simulink model "part2_MAIN"  (R2023b)
settings: Solver=FixedStepAuto  StartTime=0.0  StopTime=300  FixedStep=0.1  RelTol=1e-3
values from neighbouring files (symbols this model uses):
  Af = diag(ti)    [init.m]
  Aw = [zeros(3) eye(3) ... (first row only)    [get_observer_parameters.m]
  B = [zeros(6,3);zeros(3,3);zeros(3,3);inv(M)]    [get_observer_parameters.m]
  change_position_time = 1200    [init.m]
  Cw = [zeros(3) eye(3)]    [get_observer_parameters.m]
  D = Damping    [init.m]
  Damping = diag([2.6486e5, 8.8164e5, 3.3774e8])    [init.m]
  direction_limit = pi/36    (= 0.0872664625997)    [init.m]
  direction_time_constant = 100    [init.m]
  dt = 0.1    [get_observer_parameters.m]
  E = [Ew, zeros(6,3) ... (first row only)    [get_observer_parameters.m]
  Gamma = diag(omega_is)    [init.m]
  gust_limit = 40    [init.m]
  H = [Cw, eye(3), zeros(3,3) zeros(3,3)]    [get_observer_parameters.m]
  height = 3    [init.m]
  inv_M = inv(M)    [get_observer_parameters.m]
  inv_Tb = inv(Tb)    [get_observer_parameters.m]
  kappa = 0.003    [init.m]
  kappa2 = 0.0026    [init.m]
  Kd = [1660451.40544401; 3920391.80535684; 1605063439.04156]    [init.m]
  Ki = [137.081306245593; 3163.274947400198; 335358.448218978]    [init.m]
  Kp = [75459.3345349083; 277551.73586971; 120744473.878042]    [init.m]
  L = 1800    [init.m]
  M = Mass    [init.m]
  mean_wind_direction = pi    (= 3.14159265359)    [init.m]
  observer_type = 0    [init.m]
  Omega = diag([omega_n])    [get_observer_parameters.m]    (also in init.m = diag(2*omega_is.*zeta_is))
  Q = diag([0.1,0.1,pi/180,1e6,1e6,1e9])*10e3    [get_observer_parameters.m]
  R = diag([0.00001,0.00001,0.01*pi/180])*10e-4    [get_observer_parameters.m]
  simu_step = 36    [init.m]
  simulation = 5    [init.m]
  slow_varying_limit = 1    [init.m]
  slow_varying_time_constant = 100    [init.m]
  TAU = dt*E    [get_observer_parameters.m]
  Tb = 0.1 * eye(3)    [get_observer_parameters.m]
  thruster_type = 0    [init.m]
  u10 = 12    [init.m]
  wind = 1    [init.m]
  x_current = u_c*cos(xi)    [init.m]
  y_current = u_c*sin(xi)    [init.m]
undefined symbols (not defined in the file or in its folder): Hoerner, ModelParams, npf, Param, thrusters, vessel, WaveModel
libraries: dspsigops x42, simulink x30, marine_hydro x16, marine_gnc x8, slpidlib x3
(part 8 of 8)

== matlab function part2_MAIN/Simulation 7/Observer/EKF/MATLAB Function ==
  data: y input; U input; P input; P_update output; states input; states_update output; states_hat output; error output; M input; D input; inv_M input; Aw input; Tb input; Cw input; E input; B input; H input; R input; Q input; dt input; inv_Tb input; TAU input; K output
function [P_update, states_update,states_hat,error, K]= fcn(y, U, P, states,M,D,inv_M, Aw,Tb,Cw,E,B,H,R,Q,dt, inv_Tb, TAU)
%%%P - 15x15
%states [zeta,eta, b, nu] --15x1
%zeta - 6x1, 
%eta - 3x1, 
%b - 3x1, 
%nu - 3x1
%u - 3x1 force input 

%Aw, Tb, B, E, H
%%%states
zeta = states(1:6,:);
eta = states(7:9,:);
b = states(10:12,:);
nu = states(13:15,:);

u = nu(1,1);
v = nu(2,1);
b_x = b(1,1);
b_y = b(2,1);


%% calculating FXU

Rot_R = [cos(eta(3,1)) -sin(eta(3,1)) 0;
    sin(eta(3,1)) cos(eta(3,1)) 0;
    0 0 1];

Fx = [
Aw*zeta;
Rot_R*nu;
-inv_Tb*b;
% zeros(3,1);
-inv_M*D*nu + inv_M*Rot_R'*b
];

F = zeros(15,1);
F = (B*U);
F = Fx +F;


%%

%predictor
%%phi = PHI(states,ws_var.dt, ws_var);
%calculating phi
A = zeros(15,15);
psi = eta(3,1);

% A(7,9) = -v*cos(psi)-u*sin(psi);
% A(7,13) = cos(psi);
% A(1,15) = 0;
% A(1,4) = 1;
% A(2,5) = 1;
% A(3,6) = 1;
% A(4,1) = -0.0987;
% A(4,4) = -0.0628;
% A(5,2) = -0.0987;
% A(5,5) = -0.0628;
% A(6,3) = -0.0987;
% A(6,6) = -0.0628;
% A(7,14) = -sin(psi);
% 
% A(8,9) = u*cos(psi)-v*sin(psi);
% A(8,13) = sin(psi);
% A(8,14) = cos(psi);
% A(9,15) = 1;
% A(10:12, 10:12) = -10*eye(3);
% A(13,9) = -1.43e-7*(b_y*cos(psi)+b_x*sin(psi));
% A(13,10) = 1.43e-7*cos(psi);
% A(13,11) = -1.43e-7*sin(psi);
% 
% A(14,9) = 1.17e-7*(b_x*cos(psi) - b_y*sin(psi));
% A(14,10) = 1.17e-7*sin(psi);
% A(14,11) = -1.46e-11;
% A(14,12) = 2.63e-10;
% 
% A(15,9) = 1.46e-11*(b_y*sin(psi) - b_x*cos(psi));
% A(15,10) = -1.46e-11*sin(psi);
% A(15,11) = -1.46e-11*cos(psi);
% A(15,12) = 2.63e-10;
% A(13:15,13:15) = -inv_M*D;
% 
A = [Aw zeros(6,9);
    zeros(3,12) Rot_R;
    zeros(3,9) -inv_Tb zeros(3,3);
    zeros(3,6) zeros(3,3) -inv_M*Rot_R' -inv_M*D];

phi = eye(15)+dt*A;
%%

% TAU = dt*E;
P_hat = phi*P*phi' + TAU*Q*TAU';
states_hat = states+dt*F;


%corrector
%kalman gain
K = P_hat*H'/(H*P_hat*H'+R);
% K = zeros(15,3);
P_update = (eye(15)-K*H)*P_hat*(eye(15)-K*H)' + K*R*K';
states_update = states_hat + K*(y-H*states_hat);
error = y - H*states_hat;
end

== matlab function part2_MAIN/ Original/Observer/Passive Non-Linear/R_psi ==
  data: u input; y output
function y = fcn(u)

rot = [cos(u) -sin(u) 0;
    sin(u) cos(u) 0;
    0 0 1];

y = rot;

== matlab function part2_MAIN/Simulation 7/Observer/EKF/MATLAB Function1 ==
  data: states_vector input; eta_hat output; nu_hat output
function [eta_hat, nu_hat] = fcn(states_vector)
%%states [zeta,eta, b, nu] --15x1
%zeta - 6x1, 
%eta - 3x1, 
%b - 3x1, 
%nu - 3x1
eta_hat = states_vector(7:9,1);
nu_hat = states_vector(13:15,1);

end

== matlab function part2_MAIN/Simulation 7/Observer/EKF/Subsystem1/MATLAB Function ==
  data: u input; P1 output; P input; states input; states1 output
function [P1, states1] = fcn(u, P, states)

if u>1
    P1 = eye(15);
    states1 = zeros(15,1);
else
    P1 = P;
    states1 = states;
end

== matlab function part2_MAIN/Simulation 7/Observer/Passive Non-Linear/R_psi ==
  data: u input; y output
function y = fcn(u)

rot = [cos(u) -sin(u) 0;
    sin(u) cos(u) 0;
    0 0 1];

y = rot;

== matlab function part2_MAIN/Simulation 7/Observer/Passive Non-Linear/R_psi_T ==
  data: u input; y output
function y = fcn(u)

rot = [cos(u) -sin(u) 0;
    sin(u) cos(u) 0;
    0 0 1];

y = rot';

== matlab function part2_MAIN/Simulation 7/Thrust Allocation/0 ==
  data: tau_d input; Td output; alpha output
function [Td, alpha] = quad_prog_basic_slow(tau_d)
%% x, y, and psi component of tau_d
tau = [tau_d(1); tau_d(2); tau_d(6)]; 

%% Quadratic Programming
% Compute function arguments
% Point to Minimize
u_p = [0 0 0 0 0 0 0 0].'; % [T1 T2x T2y T3 T4x T4y T5x T5y]
u_m = -[0 0 0 0 0 0 0 0].'; % [T1 T2x T2y T3 T4x T4y T5x T5y]
s_p = [0 0 0].'; % [x1 x2 x6]
s_m = -[0 0 0].'; % [x1 x2 x6]
x0 = [u_p; u_m; s_p; s_m]; % auxiliary variables

% persistent x0_l
% 
% % Store previous point
% if isempty(x0_l)
%     x0_l = x0(1:16);
% end

% Objective Function
% Quadratic Objective Term
sWeight = 1e4;
w = [1 1 1 1 0.8 0.8 0.8 0.8]; % Prioritize control over T4 and T5
q = [sWeight sWeight sWeight*10]; % For slackness (Needs Tuning)
H = 2*diag([w w q q]);

% Linear Objective Term
% f = zeros(1, length(x0)); % No linear term in the objective function
f = [];

% Thruster Equality Constraints
% Thruster 1
x1 = 39.3;
y1 = 0;
% Thruster 2
x2 = 35.6;
y2 = 0;
% Thruster 3
x3 = 31.3;
y3 = 0;
% Thruster 4
x4 = -28.5;
y4 = 5;
% Thruster 5
x5 = -28.5;
y5 = -5;

% Redistributed force for each thruster
thr1 = [0 1 x1].';
thr2_x = [1 0 y2].';
thr2_y = [0 1 x2].';
thr3 = [0 1 x3].';
thr4_x = [1 0 y4].';
thr4_y = [0 1 x4].';
thr5_x = [1 0 y5].';
thr5_y = [0 1 x5].';

% B redistributed
B_r = [thr1 thr2_x thr2_y thr3 thr4_x thr4_y thr5_x thr5_y];

Aeq = [B_r -B_r eye(3) -eye(3)];
beq = tau;

% Thruster Saturation Constraints
u_max = [125000, 150000, 150000, 125000, 300000, 300000, 300000, 300000].';
% u_min = [-125000 0 0 -125000 0 0 0 0].';
u_min = -u_max;

% Rate Limitation Constraints
timestep = 0.1;
delta_max = [125000/8*timestep, 150000/8*timestep, 150000/8*timestep, 125000/8*timestep, 300000/10*timestep, 300000/10*timestep, 300000/10*timestep, 300000/10*timestep];
delta_min = -delta_max;

% lim_max = delta_max - x0_l;
% lim_min = delta_min + x0_l;

A = [eye(8) -eye(8) zeros(8,3) zeros(8,3);
     -eye(8) eye(8) zeros(8,3) zeros(8,3)];

% b = [-(max(u_min, lim_min));
%      min(u_max, lim_max)];
b = [-u_min;
    u_max];

lb = [];
ub = [];

options = optimoptions('quadprog', 'Algorithm', 'active-set');

% Compute optimal thruster control
x0_opt = quadprog(H,f,A,b,Aeq,beq,lb,ub,x0, options);

% % Store previous x0_opt
% x0_l = x0_opt(1:16);

% Slack Variable from auxiliary variables
s = x0_opt(17:19) - x0_opt(20:22); % STILL DON'T NOW WHAT TO DO WITH THIS
s_abs = x0_opt(17:19) + x0_opt(20:22); % STILL DON'T NOW WHAT TO DO WITH THIS

% Allocation variables from auxiliary variables
u = x0_opt(1:8) - x0_opt(9:16); 
u_abs = x0_opt(1:8) + x0_opt(9:16); 

%% RESULTS
% Thruster control
Td = [u(1); 
      sqrt(u(2)^2 + u(3)^2); 
      u(4); 
      sqrt(u(5)^2 + u(6)^2);
      sqrt(u(7)^2 + u(8)^2)];

% Thruster angle
alpha2 = atan2(u(3),u(2));
alpha4 = atan2(u(6),u(5));
alpha5 = atan2(u(8),u(7));
alpha = [pi/2; alpha2; pi/2; alpha4; alpha5];
end
% function [Td, alpha] = quad_prog_basic(tau_d)
% %% x, y, and psi component of tau_d
% tau = [tau_d(1); tau_d(2); tau_d(6)]; 
% 
% %% Quadratic Programming
% % Compute function arguments
% % Point to Minimize
% u = [0 0 0 0 0 0 0 0].'; % [T1 T2x T2y T3 T4x T4y T5x T5y]
% s = [0 0 0].'; % [x1 x2 x6]
% x0 = [u; s]; % auxiliary variables
% 
% % persistent x0_l
% % 
% % if isempty(x0_l)
% %     x0_l = x0;
% % end
% 
% % Objective Function
% % Quadratic Objective Term
% sWeight = 1e4;
% w = [1 1 1 1 0.8 0.8 0.8 0.8]; % Prioritize control over T4 and T5
% q = [sWeight sWeight sWeight*10]; % For slackness (Needs Tuning)
% H = 2*diag([w q]);
% 
% % Linear Objective Term
% f = zeros(length(x0),1); % No linear term in the objective function 
% % f = [];
% 
% % Thruster Equality Constraints
% % Thruster 1
% x1 = 39.3;
% y1 = 0;
% % Thruster 2
% x2 = 35.6;
% y2 = 0;
% % Thruster 3
% x3 = 31.3;
% y3 = 0;
% % Thruster 4
% x4 = -28.5;
% y4 = 5;
% % Thruster 5
% x5 = -28.5;
% y5 = -5;
% 
% % Redistributed force for each thruster
% thr1 = [0 1 x1].';
% thr2_x = [1 0 y2].';
% thr2_y = [0 1 x2].';
% thr3 = [0 1 x3].';
% thr4_x = [1 0 y4].';
% thr4_y = [0 1 x4].';
% thr5_x = [1 0 y5].';
% thr5_y = [0 1 x5].';
% 
% % B redistributed
% B_r = [thr1 thr2_x thr2_y thr3 thr4_x thr4_y thr5_x thr5_y];
% 
% Aeq = [B_r, -eye(3)];
% beq = tau;
% 
% % Thruster Saturation Constraints
% u_max = [125000 150000 150000 125000 300000 300000 300000 300000].';
% u_min = -u_max;
% % u_min = [-125000 0 0 -125000 0 0 0 0].';
% 
% A = [-eye(8), zeros(8,3);
%      eye(8), zeros(8,3)];
% 
% b = [-u_min;
%      u_max];
% 
% % coder.extrinsic('quadprog');
% % coder.extrinsic('optimoptions');
% % options = optimoptions('quadprog','Algorithm','interior-point-convex','Display','off','Steptolerance',1e-30,'OptimalityTolerance',1e+3);
% options = optimoptions('quadprog', 'Algorithm', 'active-set');
% % options = optimoptions('quadprog', 'Algorithm', 'interior-point-convex', 'Display', 'iter');
% 
% % Compute optimal thruster control\
% x0_opt = quadprog(H,f,A,b,Aeq,beq,[],[],x0,options);
% 
% % Store previous x0_opt
% % x0_l = x0_opt;
% 
% % Allocation variables from auxiliary variables
% u_f = x0_opt(1:8); 
% 
% %% RESULTS
% % Thruster control
% Td = [u_f(1); 
%       sqrt(u_f(2)^2 + u_f(3)^2); 
%       u_f(4); 
%       sqrt(u_f(5)^2 + u_f(6)^2);
%       sqrt(u_f(7)^2 + u_f(8)^2)];
% 
% % Thruster angle
% alpha2 = atan2(u_f(3),u_f(2));
% alpha4 = atan2(u_f(6),u_f(5));
% alpha5 = atan2(u_f(8),u_f(7));
% alpha = [pi/2; alpha2; pi/2; alpha4; alpha5];
% end

== matlab function part2_MAIN/Simulation 7/Thrust Allocation/1 ==
  data: tau_d input; Td output; alpha output
function [Td, alpha] = p_inv_B(tau_d)
%% Build the B matrix
% Thruster 1
x1 = 39.3;
y1 = 0;
% Thruster 2
x2 = 35.6;
y2 = 0;
% Thruster 3
x3 = 31.3;
y3 = 0;
% Thruster 4
x4 = -28.5;
y4 = 5;
% Thruster 5
x5 = -28.5;
y5 = -5;

% Redistributed force for each thruster
thr1 = [0 1 x1].';
thr2_x = [1 0 y2].';
thr2_y = [0 1 x2].';
thr3 = [0 1 x3].';
thr4_x = [1 0 y4].';
thr4_y = [0 1 x4].';
thr5_x = [1 0 y5].';
thr5_y = [0 1 x5].';

% B redistributed
B = [thr1 thr2_x thr2_y thr3 thr4_x thr4_y thr5_x thr5_y];

%% Result
tau = [tau_d(1); tau_d(2); tau_d(6)];

Td_r = pinv(B) * tau;

% Thruster control
Td = [Td_r(1); 
      sqrt(Td_r(2)^2 + Td_r(3)^2); 
      Td_r(4); 
      sqrt(Td_r(5)^2 + Td_r(6)^2);
      sqrt(Td_r(7)^2 + Td_r(8)^2)];

% Thruster angle
% if Td_r(2) == 0
%     alpha2 = pi/2;
% else
%     alpha2 = atan(Td_r(3)/Td_r(2));
% end
% if Td_r(5) == 0
%     alpha4 = pi/2;
% else
%     alpha4 = atan(Td_r(6)/Td_r(5));
% end
% if Td_r(7) == 0
%     alpha5 = pi/2;
% else
%     alpha5 = atan(Td_r(8)/Td_r(7));
% end

alpha2 = atan2(Td_r(3),Td_r(2));
alpha4 = atan2(Td_r(6),Td_r(5));
alpha5 = atan2(Td_r(8),Td_r(7));

%atan2(num,den)

% alpha2 = atan(Td_r(3)/Td_r(2));
% alpha4 = atan(Td_r(6)/Td_r(5));
% alpha5 = atan(Td_r(8)/Td_r(7));

alpha = [pi/2; alpha2; pi/2; alpha4; alpha5];
end

== matlab function part2_MAIN/Simulation 7/Thruster Dynamics/MATLAB Function ==
  data: alpha_actual input; thrust_actual input; actual_tau output; PosX input; PosY input
function actual_tau   = fcn(alpha_actual,thrust_actual,PosX,PosY)

    Alpha_surge =[cos(alpha_actual(1)) cos(alpha_actual(2)) cos(alpha_actual(3)) cos(alpha_actual(4)) cos(alpha_actual(5))];  
    Alpha_sway = [sin(alpha_actual(1)) sin(alpha_actual(2)) sin(alpha_actual(3)) sin(alpha_actual(4)) sin(alpha_actual(5))];
    Alpha_yaw = [sin(alpha_actual(1))*PosX(1)-cos(alpha_actual(1))*PosY(1) sin(alpha_actual(2))*PosX(2)-cos(alpha_actual(2))*PosY(2) ...
                 sin(alpha_actual(3))*PosX(3)-cos(alpha_actual(3))*PosY(3) sin(alpha_actual(4))*PosX(4)-cos(alpha_actual(4))*PosY(4) ...
                 sin(alpha_actual(5))*PosX(5)-cos(alpha_actual(5))*PosY(5)];

    actual_tau = [Alpha_surge; Alpha_sway; Alpha_yaw]*thrust_actual;
end

== matlab function part2_MAIN/ Original/Thrust Allocation/MATLAB Function ==
  data: tau_d input; Td output; alpha output
function [Td, alpha] = p_inv_B(tau_d)
%% Build the B matrix
% Thruster 1
x1 = 39.3;
y1 = 0;
% Thruster 2
x2 = 35.6;
y2 = 0;
% Thruster 3
x3 = 31.3;
y3 = 0;
% Thruster 4
x4 = -28.5;
y4 = 5;
% Thruster 5
x5 = -28.5;
y5 = -5;

% Redistributed force for each thruster
thr1 = [0 1 x1].';
thr2_x = [1 0 y2].';
thr2_y = [0 1 x2].';
thr3 = [0 1 x3].';
thr4_x = [1 0 y4].';
thr4_y = [0 1 x4].';
thr5_x = [1 0 y5].';
thr5_y = [0 1 x5].';

% B redistributed
B = [thr1 thr2_x thr2_y thr3 thr4_x thr4_y thr5_x thr5_y];

%% Result
tau = [tau_d(1); tau_d(2); tau_d(6)];

Td_r = pinv(B) * tau;

% Thruster control
Td = [Td_r(1); 
      sqrt(Td_r(2)^2 + Td_r(3)^2); 
      Td_r(4); 
      sqrt(Td_r(5)^2 + Td_r(6)^2);
      sqrt(Td_r(7)^2 + Td_r(8)^2)];

% Thruster angle
% if Td_r(2) == 0
%     alpha2 = pi/2;
% else
%     alpha2 = atan(Td_r(3)/Td_r(2));
% end
% if Td_r(5) == 0
%     alpha4 = pi/2;
% else
%     alpha4 = atan(Td_r(6)/Td_r(5));
% end
% if Td_r(7) == 0
%     alpha5 = pi/2;
% else
%     alpha5 = atan(Td_r(8)/Td_r(7));
% end

alpha2 = atan2(Td_r(3),Td_r(2));
alpha4 = atan2(Td_r(6),Td_r(5));
alpha5 = atan2(Td_r(8),Td_r(7));

%atan2(num,den)

% alpha2 = atan(Td_r(3)/Td_r(2));
% alpha4 = atan(Td_r(6)/Td_r(5));
% alpha5 = atan(Td_r(8)/Td_r(7));

alpha = [pi/2; alpha2; pi/2; alpha4; alpha5];
end

== matlab function part2_MAIN/Simulation 7/Wind/V_w1/Gust ==
  settings: updateMethod=DISCRETE
  data: time input; u10 input; L input; kappa2 input; gust output
function gust = fcn(time, u10, L, kappa2)

nfreq = 100;
phases = 2*pi * rand(nfreq,1);
gust_tot = 0;
f = zeros(1, nfreq);

for i = 1:nfreq
    f(i) = 0.01 + (i-1)/(nfreq-1) * 0.99;
    f_tilde = L*f(i)/u10;
    S = (4*kappa2*L*u10)/((2+f_tilde^2)^(5/6));
    df = abs(f(2) - f(1));
    gust_part = sqrt(2*S*df)*cos(2*pi*f(i)*time + phases(i));
    gust_tot = gust_tot + gust_part;
end

gust = gust_tot;

== matlab function part2_MAIN/Simulation 7/Wind/V_w1/Mean wind component ==
  data: u10 input; mean_wind output; kappa input; height input
function mean_wind = fcn(u10, kappa, height)
z0 = 10*exp(-2/(5*sqrt(kappa)));
mean_wind = u10 * (5/2) * sqrt(kappa)*log(height/z0);

== matlab function part2_MAIN/Simulation 7/Wind/Wind coefficient matrix selector ==
  data: y output; angle input
function y = fcn(angle)

wind_coeff = [
  0  248.3700 0 0 0 -2355.232759 0
 10  265.1900 61.332 0 275.994 -2514.732759 551.1
 20  224.1300 136.22 0 612.99 -2125.37069 661.56
 30  149.0300 238.76 0 1074.42 -1413.215517 451.37
 40  134.3600 319.42 0 1437.39 -1274.103448 212.51
 50   96.8000 380.5 0 1712.25 -917.9310345 -23.578
 60   41.3640 396.1 0 1782.45 -392.2448276 1168.3
 70   16.4770 372.96 0 1678.32 -156.2474138 2376.3
 80    0.30412 376.5 0 1694.25 -2.883896552 3511.9
 90   -3.7230 390.01 0 1755.045 35.30431034 4610.4
100  -24.8790 386.63 0 1739.835 235.9215517 4769.5
110  -61.2810 393.76 0 1771.92 581.112931 5921.9
120 -108.5000 408.66 0 1838.97 1028.87931 6542.8
130 -169.3500 393.26 0 1769.67 1605.905172 6805.2
140 -206.6300 276.93 0 1246.185 1959.422414 6751.5
150 -201.9900 200.64 0 902.88 1915.422414 6190.1
160 -196.5100 124.71 0 561.195 1863.456897 3758.8
170 -181.5300 56.27 0 253.215 1721.405172 1905.6
180 -208.2200 0 0 0 1974.5 0
190 -181.5300 -56.27 0 -253.215 1721.405172 -1905.6
200 -196.5100 -124.71 0 -561.195 1863.456897 -3758.8
210 -201.9900 -200.64 0 -902.88 1915.422414 -6190.1
220 -206.6300 -276.93 0 -1246.185 1959.422414 -6751.5
230 -169.3500 -393.26 0 -1769.67 1605.905172 -6805.2
240 -108.5000 -408.66 0 -1838.97 1028.87931 -6542.8
250  -61.2810 -393.76 0 -1771.92 581.112931 -5921.9
260  -24.8790 -386.63 0 -1739.835 235.9215517 -4769.5
270  -3.72300 -390.01 0 -1755.045 35.30431034 -4610.4
280   0.30412 -376.5 0 -1694.25 -2.883896552 -3511.9
290  16.47700 -372.96 0 -1678.32 -156.2474138 -2376.3
300  41.36400 -396.1 0 -1782.45 -392.2448276 -1168.3
310  96.80000 -380.5 0 -1712.25 -917.9310345 23.578
320  134.3600 -319.42 0 -1437.39 -1274.103448 -212.51
330  149.0300 -238.76 0 -1074.42 -1413.215517 -451.37
340  224.1300 -136.22 0 -612.99 -2125.37069 -661.56
350  265.1900 -61.332 0 -275.994 -2514.732759 -551.1
360  248.3700 0 0 0 -2355.232759 0];

angle = abs(angle);

angle = (180/pi)*angle;

if angle > 360
    angle = angle - 360;
end



angle = int32(angle);

angle = int32(10*floor(angle/10));

i = 1;
j = 1;

while j < 38
    if int32(wind_coeff(j,1)) == angle
        i = j;
    end
    j = j+1;
end
y = wind_coeff(i,:);

== matlab function part2_MAIN/Simulation 1/Current (North - East)/MATLAB Function ==
  data: u input; y output
function y = fcn(u)
rot = [cos(u) -sin(u) 0;
    sin(u) cos(u) 0;
    0 0 1];

y = rot';

== matlab function part2_MAIN/Simulation 1/DP Controller/MATLAB Function ==
  data: u input; y output
function y = fcn(u)

rot = [cos(u) -sin(u) 0;
    sin(u) cos(u) 0;
    0 0 1];

y = rot';

== matlab function part2_MAIN/Simulation 1/DP Controller/MATLAB Function1 ==
  data: u input; y output
function y = fcn(u)

rot = [cos(u) -sin(u) 0;
    sin(u) cos(u) 0;
    0 0 1];

y = rot';

== matlab function part2_MAIN/Simulation 1/Observer/EKF/MATLAB Function ==
  data: y input; U input; P input; P_update output; states input; states_update output; states_hat output; error output; M input; D input; inv_M input; Aw input; Tb input; Cw input; E input; B input; H input; R input; Q input; dt input; inv_Tb input; TAU input; K output
function [P_update, states_update,states_hat,error, K]= fcn(y, U, P, states,M,D,inv_M, Aw,Tb,Cw,E,B,H,R,Q,dt, inv_Tb, TAU)
%%%P - 15x15
%states [zeta,eta, b, nu] --15x1
%zeta - 6x1, 
%eta - 3x1, 
%b - 3x1, 
%nu - 3x1
%u - 3x1 force input 

%Aw, Tb, B, E, H
%%%states
zeta = states(1:6,:);
eta = states(7:9,:);
b = states(10:12,:);
nu = states(13:15,:);

u = nu(1,1);
v = nu(2,1);
b_x = b(1,1);
b_y = b(2,1);


%% calculating FXU

Rot_R = [cos(eta(3,1)) -sin(eta(3,1)) 0;
    sin(eta(3,1)) cos(eta(3,1)) 0;
    0 0 1];

Fx = [
Aw*zeta;
Rot_R*nu;
-inv_Tb*b;
% zeros(3,1);
-inv_M*D*nu + inv_M*Rot_R'*b
];

F = zeros(15,1);
F = (B*U);
F = Fx +F;


%%

%predictor
%%phi = PHI(states,ws_var.dt, ws_var);
%calculating phi
A = zeros(15,15);
psi = eta(3,1);

% A(7,9) = -v*cos(psi)-u*sin(psi);
% A(7,13) = cos(psi);
% A(1,15) = 0;
% A(1,4) = 1;
% A(2,5) = 1;
% A(3,6) = 1;
% A(4,1) = -0.0987;
% A(4,4) = -0.0628;
% A(5,2) = -0.0987;
% A(5,5) = -0.0628;
% A(6,3) = -0.0987;
% A(6,6) = -0.0628;
% A(7,14) = -sin(psi);
% 
% A(8,9) = u*cos(psi)-v*sin(psi);
% A(8,13) = sin(psi);
% A(8,14) = cos(psi);
% A(9,15) = 1;
% A(10:12, 10:12) = -10*eye(3);
% A(13,9) = -1.43e-7*(b_y*cos(psi)+b_x*sin(psi));
% A(13,10) = 1.43e-7*cos(psi);
% A(13,11) = -1.43e-7*sin(psi);
% 
% A(14,9) = 1.17e-7*(b_x*cos(psi) - b_y*sin(psi));
% A(14,10) = 1.17e-7*sin(psi);
% A(14,11) = -1.46e-11;
% A(14,12) = 2.63e-10;
% 
% A(15,9) = 1.46e-11*(b_y*sin(psi) - b_x*cos(psi));
% A(15,10) = -1.46e-11*sin(psi);
% A(15,11) = -1.46e-11*cos(psi);
% A(15,12) = 2.63e-10;
% A(13:15,13:15) = -inv_M*D;
% 
A = [Aw zeros(6,9);
    zeros(3,12) Rot_R;
    zeros(3,9) -inv_Tb zeros(3,3);
    zeros(3,6) zeros(3,3) -inv_M*Rot_R' -inv_M*D];

phi = eye(15)+dt*A;
%%

% TAU = dt*E;
P_hat = phi*P*phi' + TAU*Q*TAU';
states_hat = states+dt*F;


%corrector
%kalman gain
K = P_hat*H'/(H*P_hat*H'+R);
% K = zeros(15,3);
P_update = (eye(15)-K*H)*P_hat*(eye(15)-K*H)' + K*R*K';
states_update = states_hat + K*(y-H*states_hat);
error = y - H*states_hat;
end

== matlab function part2_MAIN/ Original/Observer/EKF/MATLAB Function ==
  data: y input; U input; P input; P_update output; states input; states_update output; states_hat output; error output; M input; D input; inv_M input; Aw input; Tb input; Cw input; E input; B input; H input; R input; Q input; dt input; inv_Tb input; TAU input; K output
function [P_update, states_update,states_hat,error, K]= fcn(y, U, P, states,M,D,inv_M, Aw,Tb,Cw,E,B,H,R,Q,dt, inv_Tb, TAU)
%%%P - 15x15
%states [zeta,eta, b, nu] --15x1
%zeta - 6x1, 
%eta - 3x1, 
%b - 3x1, 
%nu - 3x1
%u - 3x1 force input 

%Aw, Tb, B, E, H
%%%states
zeta = states(1:6,:);
eta = states(7:9,:);
b = states(10:12,:);
nu = states(13:15,:);

u = nu(1,1);
v = nu(2,1);
b_x = b(1,1);
b_y = b(2,1);


%% calculating FXU

Rot_R = [cos(eta(3,1)) -sin(eta(3,1)) 0;
    sin(eta(3,1)) cos(eta(3,1)) 0;
    0 0 1];

Fx = [
Aw*zeta;
Rot_R*nu;
-inv_Tb*b;
% zeros(3,1);
-inv_M*D*nu + inv_M*Rot_R'*b
];

F = zeros(15,1);
F = (B*U);
F = Fx +F;


%%

%predictor
%%phi = PHI(states,ws_var.dt, ws_var);
%calculating phi
A = zeros(15,15);
psi = eta(3,1);

% A(7,9) = -v*cos(psi)-u*sin(psi);
% A(7,13) = cos(psi);
% A(1,15) = 0;
% A(1,4) = 1;
% A(2,5) = 1;
% A(3,6) = 1;
% A(4,1) = -0.0987;
% A(4,4) = -0.0628;
% A(5,2) = -0.0987;
% A(5,5) = -0.0628;
% A(6,3) = -0.0987;
% A(6,6) = -0.0628;
% A(7,14) = -sin(psi);
% 
% A(8,9) = u*cos(psi)-v*sin(psi);
% A(8,13) = sin(psi);
% A(8,14) = cos(psi);
% A(9,15) = 1;
% A(10:12, 10:12) = -10*eye(3);
% A(13,9) = -1.43e-7*(b_y*cos(psi)+b_x*sin(psi));
% A(13,10) = 1.43e-7*cos(psi);
% A(13,11) = -1.43e-7*sin(psi);
% 
% A(14,9) = 1.17e-7*(b_x*cos(psi) - b_y*sin(psi));
% A(14,10) = 1.17e-7*sin(psi);
% A(14,11) = -1.46e-11;
% A(14,12) = 2.63e-10;
% 
% A(15,9) = 1.46e-11*(b_y*sin(psi) - b_x*cos(psi));
% A(15,10) = -1.46e-11*sin(psi);
% A(15,11) = -1.46e-11*cos(psi);
% A(15,12) = 2.63e-10;
% A(13:15,13:15) = -inv_M*D;
% 
A = [Aw zeros(6,9);
    zeros(3,12) Rot_R;
    zeros(3,9) -inv_Tb zeros(3,3);
    zeros(3,6) zeros(3,3) -inv_M*Rot_R' -inv_M*D];

phi = eye(15)+dt*A;
%%

% TAU = dt*E;
P_hat = phi*P*phi' + TAU*Q*TAU';
states_hat = states+dt*F;


%corrector
%kalman gain
K = P_hat*H'/(H*P_hat*H'+R);
% K = zeros(15,3);
P_update = (eye(15)-K*H)*P_hat*(eye(15)-K*H)' + K*R*K';
states_update = states_hat + K*(y-H*states_hat);
error = y - H*states_hat;
end

== matlab function part2_MAIN/Simulation 1/Observer/EKF/MATLAB Function1 ==
  data: states_vector input; eta_hat output; nu_hat output
function [eta_hat, nu_hat] = fcn(states_vector)
%%states [zeta,eta, b, nu] --15x1
%zeta - 6x1, 
%eta - 3x1, 
%b - 3x1, 
%nu - 3x1
eta_hat = states_vector(7:9,1);
nu_hat = states_vector(13:15,1);

end

== matlab function part2_MAIN/Simulation 1/Observer/EKF/Subsystem1/MATLAB Function ==
  data: u input; P1 output; P input; states input; states1 output
function [P1, states1] = fcn(u, P, states)

if u>1
    P1 = eye(15);
    states1 = zeros(15,1);
else
    P1 = P;
    states1 = states;
end

== matlab function part2_MAIN/Simulation 1/Observer/Passive Non-Linear/R_psi ==
  data: u input; y output
function y = fcn(u)

rot = [cos(u) -sin(u) 0;
    sin(u) cos(u) 0;
    0 0 1];

y = rot;

== matlab function part2_MAIN/Simulation 1/Observer/Passive Non-Linear/R_psi_T ==
  data: u input; y output
function y = fcn(u)

rot = [cos(u) -sin(u) 0;
    sin(u) cos(u) 0;
    0 0 1];

y = rot';

== matlab function part2_MAIN/Simulation 1/Thrust Allocation/0 ==
  data: tau_d input; Td output; alpha output
function [Td, alpha] = quad_prog_basic_slow(tau_d)
%% x, y, and psi component of tau_d
tau = [tau_d(1); tau_d(2); tau_d(6)]; 

%% Quadratic Programming
% Compute function arguments
% Point to Minimize
u_p = [0 0 0 0 0 0 0 0].'; % [T1 T2x T2y T3 T4x T4y T5x T5y]
u_m = -[0 0 0 0 0 0 0 0].'; % [T1 T2x T2y T3 T4x T4y T5x T5y]
s_p = [0 0 0].'; % [x1 x2 x6]
s_m = -[0 0 0].'; % [x1 x2 x6]
x0 = [u_p; u_m; s_p; s_m]; % auxiliary variables

% persistent x0_l
% 
% % Store previous point
% if isempty(x0_l)
%     x0_l = x0(1:16);
% end

% Objective Function
% Quadratic Objective Term
sWeight = 1e4;
w = [1 1 1 1 0.8 0.8 0.8 0.8]; % Prioritize control over T4 and T5
q = [sWeight sWeight sWeight*10]; % For slackness (Needs Tuning)
H = 2*diag([w w q q]);

% Linear Objective Term
% f = zeros(1, length(x0)); % No linear term in the objective function
f = [];

% Thruster Equality Constraints
% Thruster 1
x1 = 39.3;
y1 = 0;
% Thruster 2
x2 = 35.6;
y2 = 0;
% Thruster 3
x3 = 31.3;
y3 = 0;
% Thruster 4
x4 = -28.5;
y4 = 5;
% Thruster 5
x5 = -28.5;
y5 = -5;

% Redistributed force for each thruster
thr1 = [0 1 x1].';
thr2_x = [1 0 y2].';
thr2_y = [0 1 x2].';
thr3 = [0 1 x3].';
thr4_x = [1 0 y4].';
thr4_y = [0 1 x4].';
thr5_x = [1 0 y5].';
thr5_y = [0 1 x5].';

% B redistributed
B_r = [thr1 thr2_x thr2_y thr3 thr4_x thr4_y thr5_x thr5_y];

Aeq = [B_r -B_r eye(3) -eye(3)];
beq = tau;

% Thruster Saturation Constraints
u_max = [125000, 150000, 150000, 125000, 300000, 300000, 300000, 300000].';
% u_min = [-125000 0 0 -125000 0 0 0 0].';
u_min = -u_max;

% Rate Limitation Constraints
timestep = 0.1;
delta_max = [125000/8*timestep, 150000/8*timestep, 150000/8*timestep, 125000/8*timestep, 300000/10*timestep, 300000/10*timestep, 300000/10*timestep, 300000/10*timestep];
delta_min = -delta_max;

% lim_max = delta_max - x0_l;
% lim_min = delta_min + x0_l;

A = [eye(8) -eye(8) zeros(8,3) zeros(8,3);
     -eye(8) eye(8) zeros(8,3) zeros(8,3)];

% b = [-(max(u_min, lim_min));
%      min(u_max, lim_max)];
b = [-u_min;
    u_max];

lb = [];
ub = [];

options = optimoptions('quadprog', 'Algorithm', 'active-set');

% Compute optimal thruster control
x0_opt = quadprog(H,f,A,b,Aeq,beq,lb,ub,x0, options);

% % Store previous x0_opt
% x0_l = x0_opt(1:16);

% Slack Variable from auxiliary variables
s = x0_opt(17:19) - x0_opt(20:22); % STILL DON'T NOW WHAT TO DO WITH THIS
s_abs = x0_opt(17:19) + x0_opt(20:22); % STILL DON'T NOW WHAT TO DO WITH THIS

% Allocation variables from auxiliary variables
u = x0_opt(1:8) - x0_opt(9:16); 
u_abs = x0_opt(1:8) + x0_opt(9:16); 

%% RESULTS
% Thruster control
Td = [u(1); 
      sqrt(u(2)^2 + u(3)^2); 
      u(4); 
      sqrt(u(5)^2 + u(6)^2);
      sqrt(u(7)^2 + u(8)^2)];

% Thruster angle
alpha2 = atan2(u(3),u(2));
alpha4 = atan2(u(6),u(5));
alpha5 = atan2(u(8),u(7));
alpha = [pi/2; alpha2; pi/2; alpha4; alpha5];
end
% function [Td, alpha] = quad_prog_basic(tau_d)
% %% x, y, and psi component of tau_d
% tau = [tau_d(1); tau_d(2); tau_d(6)]; 
% 
% %% Quadratic Programming
% % Compute function arguments
% % Point to Minimize
% u = [0 0 0 0 0 0 0 0].'; % [T1 T2x T2y T3 T4x T4y T5x T5y]
% s = [0 0 0].'; % [x1 x2 x6]
% x0 = [u; s]; % auxiliary variables
% 
% % persistent x0_l
% % 
% % if isempty(x0_l)
% %     x0_l = x0;
% % end
% 
% % Objective Function
% % Quadratic Objective Term
% sWeight = 1e4;
% w = [1 1 1 1 0.8 0.8 0.8 0.8]; % Prioritize control over T4 and T5
% q = [sWeight sWeight sWeight*10]; % For slackness (Needs Tuning)
% H = 2*diag([w q]);
% 
% % Linear Objective Term
% f = zeros(length(x0),1); % No linear term in the objective function 
% % f = [];
% 
% % Thruster Equality Constraints
% % Thruster 1
% x1 = 39.3;
% y1 = 0;
% % Thruster 2
% x2 = 35.6;
% y2 = 0;
% % Thruster 3
% x3 = 31.3;
% y3 = 0;
% % Thruster 4
% x4 = -28.5;
% y4 = 5;
% % Thruster 5
% x5 = -28.5;
% y5 = -5;
% 
% % Redistributed force for each thruster
% thr1 = [0 1 x1].';
% thr2_x = [1 0 y2].';
% thr2_y = [0 1 x2].';
% thr3 = [0 1 x3].';
% thr4_x = [1 0 y4].';
% thr4_y = [0 1 x4].';
% thr5_x = [1 0 y5].';
% thr5_y = [0 1 x5].';
% 
% % B redistributed
% B_r = [thr1 thr2_x thr2_y thr3 thr4_x thr4_y thr5_x thr5_y];
% 
% Aeq = [B_r, -eye(3)];
% beq = tau;
% 
% % Thruster Saturation Constraints
% u_max = [125000 150000 150000 125000 300000 300000 300000 300000].';
% u_min = -u_max;
% % u_min = [-125000 0 0 -125000 0 0 0 0].';
% 
% A = [-eye(8), zeros(8,3);
%      eye(8), zeros(8,3)];
% 
% b = [-u_min;
%      u_max];
% 
% % coder.extrinsic('quadprog');
% % coder.extrinsic('optimoptions');
% % options = optimoptions('quadprog','Algorithm','interior-point-convex','Display','off','Steptolerance',1e-30,'OptimalityTolerance',1e+3);
% options = optimoptions('quadprog', 'Algorithm', 'active-set');
% % options = optimoptions('quadprog', 'Algorithm', 'interior-point-convex', 'Display', 'iter');
% 
% % Compute optimal thruster control\
% x0_opt = quadprog(H,f,A,b,Aeq,beq,[],[],x0,options);
% 
% % Store previous x0_opt
% % x0_l = x0_opt;
% 
% % Allocation variables from auxiliary variables
% u_f = x0_opt(1:8); 
% 
% %% RESULTS
% % Thruster control
% Td = [u_f(1); 
%       sqrt(u_f(2)^2 + u_f(3)^2); 
%       u_f(4); 
%       sqrt(u_f(5)^2 + u_f(6)^2);
%       sqrt(u_f(7)^2 + u_f(8)^2)];
% 
% % Thruster angle
% alpha2 = atan2(u_f(3),u_f(2));
% alpha4 = atan2(u_f(6),u_f(5));
% alpha5 = atan2(u_f(8),u_f(7));
% alpha = [pi/2; alpha2; pi/2; alpha4; alpha5];
% end

== matlab function part2_MAIN/Simulation 1/Thrust Allocation/1 ==
  data: tau_d input; Td output; alpha output
function [Td, alpha] = p_inv_B(tau_d)
%% Build the B matrix
% Thruster 1
x1 = 39.3;
y1 = 0;
% Thruster 2
x2 = 35.6;
y2 = 0;
% Thruster 3
x3 = 31.3;
y3 = 0;
% Thruster 4
x4 = -28.5;
y4 = 5;
% Thruster 5
x5 = -28.5;
y5 = -5;

% Redistributed force for each thruster
thr1 = [0 1 x1].';
thr2_x = [1 0 y2].';
thr2_y = [0 1 x2].';
thr3 = [0 1 x3].';
thr4_x = [1 0 y4].';
thr4_y = [0 1 x4].';
thr5_x = [1 0 y5].';
thr5_y = [0 1 x5].';

% B redistributed
B = [thr1 thr2_x thr2_y thr3 thr4_x thr4_y thr5_x thr5_y];

%% Result
tau = [tau_d(1); tau_d(2); tau_d(6)];

Td_r = pinv(B) * tau;

% Thruster control
Td = [Td_r(1); 
      sqrt(Td_r(2)^2 + Td_r(3)^2); 
      Td_r(4); 
      sqrt(Td_r(5)^2 + Td_r(6)^2);
      sqrt(Td_r(7)^2 + Td_r(8)^2)];

% Thruster angle
% if Td_r(2) == 0
%     alpha2 = pi/2;
% else
%     alpha2 = atan(Td_r(3)/Td_r(2));
% end
% if Td_r(5) == 0
%     alpha4 = pi/2;
% else
%     alpha4 = atan(Td_r(6)/Td_r(5));
% end
% if Td_r(7) == 0
%     alpha5 = pi/2;
% else
%     alpha5 = atan(Td_r(8)/Td_r(7));
% end

alpha2 = atan2(Td_r(3),Td_r(2));
alpha4 = atan2(Td_r(6),Td_r(5));
alpha5 = atan2(Td_r(8),Td_r(7));

%atan2(num,den)

% alpha2 = atan(Td_r(3)/Td_r(2));
% alpha4 = atan(Td_r(6)/Td_r(5));
% alpha5 = atan(Td_r(8)/Td_r(7));

alpha = [pi/2; alpha2; pi/2; alpha4; alpha5];
end

== matlab function part2_MAIN/Simulation 1/Thruster Dynamics/MATLAB Function ==
  data: alpha_actual input; thrust_actual input; actual_tau output; PosX input; PosY input
function actual_tau   = fcn(alpha_actual,thrust_actual,PosX,PosY)

    Alpha_surge =[cos(alpha_actual(1)) cos(alpha_actual(2)) cos(alpha_actual(3)) cos(alpha_actual(4)) cos(alpha_actual(5))];  
    Alpha_sway = [sin(alpha_actual(1)) sin(alpha_actual(2)) sin(alpha_actual(3)) sin(alpha_actual(4)) sin(alpha_actual(5))];
    Alpha_yaw = [sin(alpha_actual(1))*PosX(1)-cos(alpha_actual(1))*PosY(1) sin(alpha_actual(2))*PosX(2)-cos(alpha_actual(2))*PosY(2) ...
                 sin(alpha_actual(3))*PosX(3)-cos(alpha_actual(3))*PosY(3) sin(alpha_actual(4))*PosX(4)-cos(alpha_actual(4))*PosY(4) ...
                 sin(alpha_actual(5))*PosX(5)-cos(alpha_actual(5))*PosY(5)];

    actual_tau = [Alpha_surge; Alpha_sway; Alpha_yaw]*thrust_actual;
end

== matlab function part2_MAIN/Simulation 1/Wind/V_w1/Gust ==
  settings: updateMethod=DISCRETE
  data: time input; u10 input; L input; kappa2 input; gust output
function gust = fcn(time, u10, L, kappa2)

nfreq = 100;
phases = 2*pi * rand(nfreq,1);
gust_tot = 0;
f = zeros(1, nfreq);

for i = 1:nfreq
    f(i) = 0.01 + (i-1)/(nfreq-1) * 0.99;
    f_tilde = L*f(i)/u10;
    S = (4*kappa2*L*u10)/((2+f_tilde^2)^(5/6));
    df = abs(f(2) - f(1));
    gust_part = sqrt(2*S*df)*cos(2*pi*f(i)*time + phases(i));
    gust_tot = gust_tot + gust_part;
end

gust = gust_tot;

== matlab function part2_MAIN/Simulation 1/Wind/V_w1/Mean wind component ==
  data: u10 input; mean_wind output; kappa input; height input
function mean_wind = fcn(u10, kappa, height)
z0 = 10*exp(-2/(5*sqrt(kappa)));
mean_wind = u10 * (5/2) * sqrt(kappa)*log(height/z0);

== matlab function part2_MAIN/Simulation 1/Wind/Wind coefficient matrix selector ==
  data: y output; angle input
function y = fcn(angle)

wind_coeff = [
  0  248.3700 0 0 0 -2355.232759 0
 10  265.1900 61.332 0 275.994 -2514.732759 551.1
 20  224.1300 136.22 0 612.99 -2125.37069 661.56
 30  149.0300 238.76 0 1074.42 -1413.215517 451.37
 40  134.3600 319.42 0 1437.39 -1274.103448 212.51
 50   96.8000 380.5 0 1712.25 -917.9310345 -23.578
 60   41.3640 396.1 0 1782.45 -392.2448276 1168.3
 70   16.4770 372.96 0 1678.32 -156.2474138 2376.3
 80    0.30412 376.5 0 1694.25 -2.883896552 3511.9
 90   -3.7230 390.01 0 1755.045 35.30431034 4610.4
100  -24.8790 386.63 0 1739.835 235.9215517 4769.5
110  -61.2810 393.76 0 1771.92 581.112931 5921.9
120 -108.5000 408.66 0 1838.97 1028.87931 6542.8
130 -169.3500 393.26 0 1769.67 1605.905172 6805.2
140 -206.6300 276.93 0 1246.185 1959.422414 6751.5
150 -201.9900 200.64 0 902.88 1915.422414 6190.1
160 -196.5100 124.71 0 561.195 1863.456897 3758.8
170 -181.5300 56.27 0 253.215 1721.405172 1905.6
180 -208.2200 0 0 0 1974.5 0
190 -181.5300 -56.27 0 -253.215 1721.405172 -1905.6
200 -196.5100 -124.71 0 -561.195 1863.456897 -3758.8
210 -201.9900 -200.64 0 -902.88 1915.422414 -6190.1
220 -206.6300 -276.93 0 -1246.185 1959.422414 -6751.5
230 -169.3500 -393.26 0 -1769.67 1605.905172 -6805.2
240 -108.5000 -408.66 0 -1838.97 1028.87931 -6542.8
250  -61.2810 -393.76 0 -1771.92 581.112931 -5921.9
260  -24.8790 -386.63 0 -1739.835 235.9215517 -4769.5
270  -3.72300 -390.01 0 -1755.045 35.30431034 -4610.4
280   0.30412 -376.5 0 -1694.25 -2.883896552 -3511.9
290  16.47700 -372.96 0 -1678.32 -156.2474138 -2376.3
300  41.36400 -396.1 0 -1782.45 -392.2448276 -1168.3
310  96.80000 -380.5 0 -1712.25 -917.9310345 23.578
320  134.3600 -319.42 0 -1437.39 -1274.103448 -212.51
330  149.0300 -238.76 0 -1074.42 -1413.215517 -451.37
340  224.1300 -136.22 0 -612.99 -2125.37069 -661.56
350  265.1900 -61.332 0 -275.994 -2514.732759 -551.1
360  248.3700 0 0 0 -2355.232759 0];

angle = abs(angle);

angle = (180/pi)*angle;

if angle > 360
    angle = angle - 360;
end



angle = int32(angle);

angle = int32(10*floor(angle/10));

i = 1;
j = 1;

while j < 38
    if int32(wind_coeff(j,1)) == angle
        i = j;
    end
    j = j+1;
end
y = wind_coeff(i,:);

== matlab function part2_MAIN/Simulation 6/Current (North - East)/MATLAB Function ==
  data: u input; y output
function y = fcn(u)
rot = [cos(u) -sin(u) 0;
    sin(u) cos(u) 0;
    0 0 1];

y = rot';

== matlab function part2_MAIN/Simulation 6/DP Controller/MATLAB Function ==
  data: u input; y output
function y = fcn(u)

rot = [cos(u) -sin(u) 0;
    sin(u) cos(u) 0;
    0 0 1];

y = rot';

== matlab function part2_MAIN/Simulation 6/DP Controller/MATLAB Function1 ==
  data: u input; y output
function y = fcn(u)

rot = [cos(u) -sin(u) 0;
    sin(u) cos(u) 0;
    0 0 1];

y = rot';
